simulink model "PFCBoost"  (R2021a)
settings: Solver=VariableStepAuto  StartTime=0.0  StopTime=1  RelTol=1e-3
libraries: spsSeriesRLCBranchLib x3, spsMosfetLib x2, spsIGBTDiodeLib x2, spsVoltageMeasurementLib x2, spsACVoltageSourceLib x1, spspowerguiLib x1
settings Model: Creator=Administrator  LastModifiedBy=Administrator

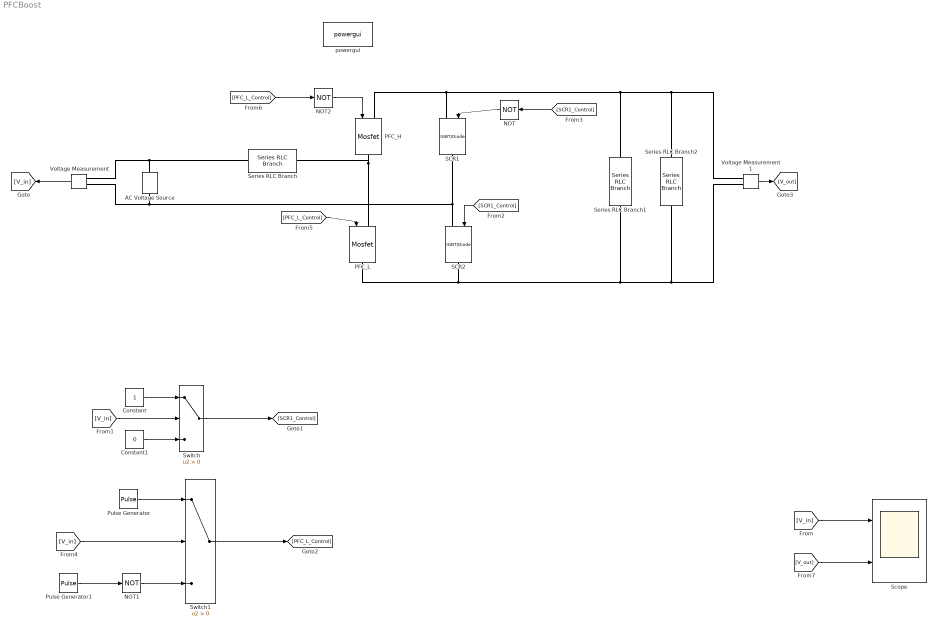
== system PFCBoost ==
  AC Voltage Source : spsACVoltageSourceLib/AC Voltage Source  Amplitude=330  Phase=0  Frequency=50  SampleTime=0  Measurements=None  BusType=swing  Pref=10e3  Qref=0  Qmin=-inf  Qmax=+inf
  Constant : Constant
  Constant1 : Constant  Value=0
  NOT : Logic  Operator=NOT  AllPortsSameDT=off  OutDataTypeStr=boolean
  NOT1 : Logic  Operator=NOT  AllPortsSameDT=off  OutDataTypeStr=boolean
  NOT2 : Logic  Operator=NOT  AllPortsSameDT=off  OutDataTypeStr=boolean
  PFC_H : spsMosfetLib/Mosfet  Ron=0.1  Lon=0  Rd=0.01  Vfd=0  IC=0  Rs=1e5  Cs=inf  Measurements=off
  PFC_L : spsMosfetLib/Mosfet  Ron=0.1  Lon=0  Rd=0.01  Vfd=0  IC=0  Rs=1e5  Cs=inf  Measurements=off
  Pulse Generator : DiscretePulseGenerator  PulseType=Time based  Period=1/100000  PulseWidth=42
  Pulse Generator1 : DiscretePulseGenerator  PulseType=Time based  Period=1/100000  PulseWidth=42
  SCR1 : spsIGBTDiodeLib/IGBT//Diode  Ron=1e-3  Rs=1e5  Cs=inf  Measurements=off
  SCR2 : spsIGBTDiodeLib/IGBT//Diode  Ron=1e-3  Rs=1e5  Cs=inf  Measurements=off
  Scope : Scope  NumInputPorts=2
  Series RLC Branch : spsSeriesRLCBranchLib/Series RLC Branch  LConnTagsString=__new0  RConnTagsString=__new0  BranchType=L  Resistance=1  Inductance=1e-3  SetiL0=off  InitialCurrent=0  Capacitance=1e-6  Setx0=off  InitialVoltage=0  Measurements=None
  Series RLC Branch1 : spsSeriesRLCBranchLib/Series RLC Branch  LConnTagsString=__new0  RConnTagsString=__new0  BranchType=C  Resistance=1  Inductance=1e-3  SetiL0=off  InitialCurrent=0  Capacitance=1e-6  Setx0=off  InitialVoltage=0  Measurements=None
  Series RLC Branch2 : spsSeriesRLCBranchLib/Series RLC Branch  LConnTagsString=__new0  RConnTagsString=__new0  BranchType=R  Resistance=100  Inductance=1e-3  SetiL0=off  InitialCurrent=0  Capacitance=1e-6  Setx0=off  InitialVoltage=0  Measurements=None
  Switch : Switch  Criteria=u2 > Threshold
  Switch1 : Switch  Criteria=u2 > Threshold
  Voltage Measurement : spsVoltageMeasurementLib/Voltage Measurement  PhasorSimulation=off  OutputType=Complex  PSBequivalent=0
  Voltage Measurement1 : spsVoltageMeasurementLib/Voltage Measurement  PhasorSimulation=off  OutputType=Complex  PSBequivalent=0
  powergui : spspowerguiLib/powergui  Priority=1  SimulationMode=Discrete  SampleTime=1/1000000  frequency=60  Iterations=50  frequencyindice=50  Pbase=100e6  ErrMax=1e-4  UnitsV=kV  UnitsW=MW  buscounter=0  FunctionMessages=off  echomessages=off  EnableUseOfTLC=off  CurrentSourceSwitches=off  DisableSnubberDevices=off  DisableRonSwitches=off  DisableVfSwitches=off  DisplayEquations=off  AutomaticDiscreteSolvers=off  SolverType=Tustin/Backward Euler (TBE)  Interpol=off  ExternalGateDelay=off  methode=off  Ts=100  x0status=blocks  SPID=on  SwTol=0  HookPort=off  NonlinearTolerance=1e-4  nMaxIteration=100  ContinueOnMaxIteration=off  RestoreLinks=warning  ResistiveCurrentMeasurement=off  Frange=[0:2:500]  Ylog=off  Xlog=on  ShowGrid=off  save=off  variable=ZData  structure=0  ZoomFFT=off  StartTime=0.0  cycles=1  DisplayStyle=1  fundamental=60  FreqAxis=off  MaxFrequency=1000  frequencyindicesteady=1  RmsSteady=1  display=off
  wires:
  Voltage Measurement/1 -> [V_in]
  [V_in] -> Scope/1
  [V_in] -> Switch/2
  Constant/1 -> Switch/1
  Constant1/1 -> Switch/3
  Switch/1 -> [SCR1_Control]
  [SCR1_Control] -> SCR2/1
  [SCR1_Control] -> NOT/1
  NOT/1 -> SCR1/1
  Pulse Generator/1 -> Switch1/1
  Pulse Generator1/1 -> NOT1/1
  [V_in] -> Switch1/2
  Switch1/1 -> [PFC_L_Control]
  NOT1/1 -> Switch1/3
  [PFC_L_Control] -> PFC_L/1
  [PFC_L_Control] -> NOT2/1
  NOT2/1 -> PFC_H/1
  Voltage Measurement1/1 -> [V_out]
  [V_out] -> Scope/2
  connections:
  AC Voltage Source/RConn1 -- Series RLC Branch/LConn1 -- Voltage Measurement/LConn1
  SCR1/LConn1 -- Series RLC Branch2/LConn1 -- Voltage Measurement1/LConn1 -- Series RLC Branch1/LConn1 -- PFC_H/LConn1
  PFC_H/RConn1 -- Series RLC Branch/RConn1 -- PFC_L/LConn1
  SCR1/RConn1 -- Voltage Measurement/LConn2 -- AC Voltage Source/LConn1 -- SCR2/LConn1
  Series RLC Branch1/RConn1 -- Voltage Measurement1/LConn2 -- Series RLC Branch2/RConn1 -- PFC_L/RConn1 -- SCR2/RConn1
